simulink model "simulink_progetto"  (R2024a)
settings: Solver=VariableStepAuto  StartTime=0.0  StopTime=10.0  RelTol=1e-3
values from neighbouring files (symbols this model uses):
  C = [0, 1]    [matlab_progetto.m]
  RR = RR_s*RR_d    [matlab_progetto.m]
  u_e = 0    [matlab_progetto.m]
  xe1 = n_s_e    (= 100)    [matlab_progetto.m]
  xe2 = n_r_e    (= 400)    [matlab_progetto.m]
libraries: simulink x2
settings Model: Creator=domenicodelgiudice  LastModifiedBy=domenicodelgiudice

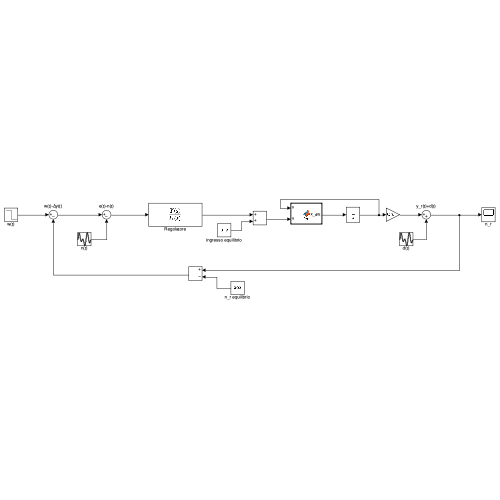
[thumbnail: Simulink's stored preview of the top-level diagram]
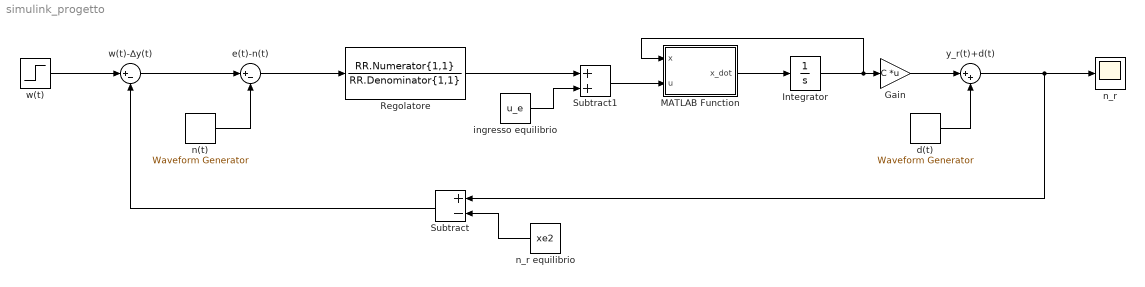
== system simulink_progetto ==
  Gain : Gain  Gain=C  Multiplication=Matrix(K*u)
  Integrator : Integrator  InitialCondition=[xe1;xe2]
  MATLAB Function : MATLAB Function  TreatAsAtomicUnit=on
  Regolatore : TransferFcn  Numerator=RR.Numerator{1,1}  Denominator=RR.Denominator{1,1}  ParameterTunability=Unconstrained  ContinuousStateAttributes='regolatore'
  Subtract : Sum  Inputs=+-
  Subtract1 : Sum
  d(t) : simulink/Sources/Waveform Generator  OutMin=[]  OutMax=[]  OutDataTypeStr=double  SelectedSignal=1  Signals=sin(-2,0.025,0)+sin(-2,0.050,0)+sin(-2,0.075,0)+sin(-2,0.1,0)  BlockNames=MultiportSwitch_75c06661c003417  SampleTime=0.0001
  e(t)-n(t) : Sum  Inputs=|+-
  ingresso equilibrio : Constant  Value=u_e
  n(t) : simulink/Sources/Waveform Generator  OutMin=[]  OutMax=[]  OutDataTypeStr=double  SelectedSignal=1  Signals=sin(0.1,5000,0)+sin(0.1,10000,0)+sin(0.1,15000,0)+sin(0.1,20000,0)  BlockNames=MultiportSwitch_6dfa9ab0c3c94a7  SampleTime=0.0001
  n_r : Scope
  n_r equilibrio : Constant  Value=xe2
  w(t) : Step  Time=0.001  After=-110  SampleTime=0.0001
  w(t)-∆y(t) : Sum  Inputs=|+-
  y_r(t)+d(t) : Sum  Inputs=|++
  wires:
  e(t)-n(t)/1 -> Regolatore/1
  Regolatore/1 -> Subtract1/1
  w(t)-∆y(t)/1 -> e(t)-n(t)/1
  y_r(t)+d(t)/1 -> Subtract/1, n_r/1
  n_r equilibrio/1 -> Subtract/2
  Subtract/1 -> w(t)-∆y(t)/2
  d(t)/1 -> y_r(t)+d(t)/2
  w(t)/1 -> w(t)-∆y(t)/1
  ingresso equilibrio/1 -> Subtract1/2
  n(t)/1 -> e(t)-n(t)/2
  MATLAB Function/1(x_dot) -> Integrator/1
  Integrator/1 -> MATLAB Function/1(x), Gain/1
  Subtract1/1 -> MATLAB Function/2(u)
  Gain/1 -> y_r(t)+d(t)/1

== matlab function simulink_progetto/MATLAB Function ==
  data: x input; u input; x_dot output
function x_dot = fcn(x,u)

r_s=1.7; %tasso riproduzione cellule suscettibili
r_r=1.4; %tasso riproduzione cellule resistenti
K=500; %num massimo cellule dell'ambiente
gamma=0.2; %costante di passaggio da r a s
beta=0.8; %costante di passaggio da s a r
alfa=0.5; %costante di mutazione a seguito del farmaco
m_s=0.95; %mortalità suscettibili
m_r=0.05; %mortalità resistenti


x_dot = zeros(2,1);
x_dot(1) = r_s * (1-(x(1)+x(2))/K) * x(1)-m_s * u * x(1)-beta * x(1)+gamma * x(2)-alfa * u * x(1);
x_dot(2) = r_r * (1-(x(1)+x(2))/K) * x(2)-m_r * u * x(2)+beta * x(1)-gamma * x(2)+alfa * u * x(1);
